simulink model "GMEKF"  (R2026b)
settings: Solver=VariableStepAuto
settings Model: Creator=mmurp  LastModifiedBy=mmurp

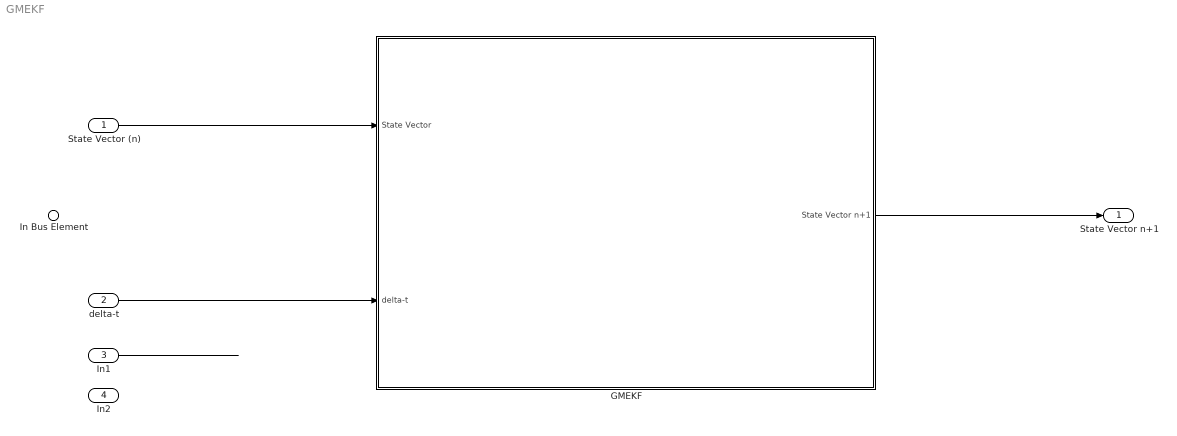
== system GMEKF ==
  State Vector (n) : Inport
  delta-t : Inport  Port=2
  In1 : Inport  Port=3
  In2 : Inport  Port=4
  In Bus Element : Inport  Port=5  PortName=InBus  Element=signal1
  GMEKF : Subsystem
  State Vector n+1 : Outport
  wires:
  State Vector (n)/1 -> GMEKF/1(State Vector)
  GMEKF/1(State Vector n+1) -> State Vector n+1/1
  delta-t/1 -> GMEKF/2(delta-t)
  In1/1 -> ?

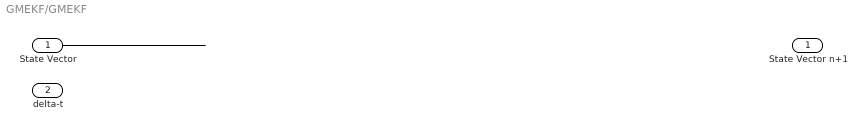
== system GMEKF/GMEKF ==
  State Vector : Inport  PortDimensions=[20 1]
  delta-t : Inport  Port=2
  State Vector n+1 : Outport
  wires:
  State Vector/1 -> ?
  ? -> State Vector n+1/1
